simulink library "discretizedSecondOrderIntegrator"  (Simulink 7.6)
settings: Solver=ode45  StartTime=0.0  StopTime=10.0  RelTol=1e-3
undefined symbols (not defined in the file or in its folder): DiscIntNeverNeededParam, LowerLimitX, UpperLimitX
libraries: simulink x28, discretizedSecondOrderIntegrator x12
settings Model: Creator=aselot  LastModifiedBy=aselot

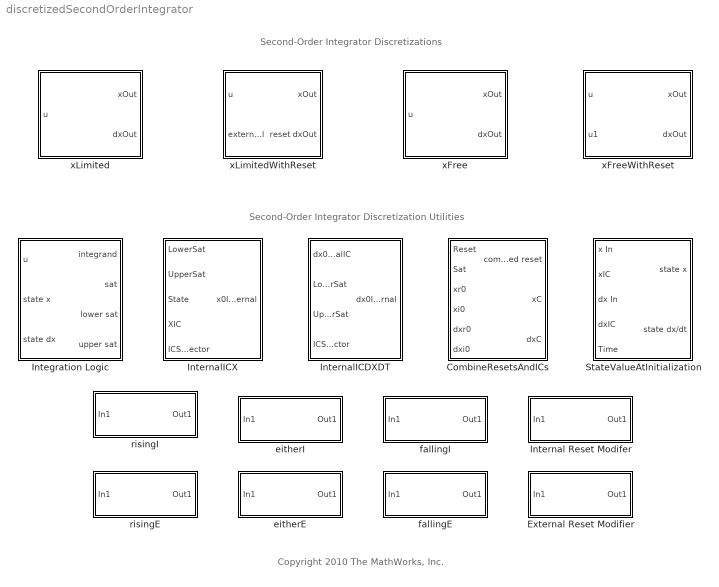
== system discretizedSecondOrderIntegrator ==
  note: Second-Order Integrator Discretizations
  note: Second-Order Integrator Discretization Utilities
  note: Copyright 2010 The MathWorks, Inc.
  CombineResetsAndICs : Subsystem
  External Reset Modifier : Subsystem  BlockChoice=risingE
      settings: TemplateBlock=self  MemberBlocks=eitherE,fallingE,risingE
  Integration Logic : Subsystem
  Internal Reset Modifer : Subsystem  BlockChoice=risingI
      settings: TemplateBlock=self  MemberBlocks=eitherI,fallingI,risingI
  InternalICDXDT : Subsystem  mask{ReinitDXDTwhenXreachesSaturation=off}
      mask prompts: ReinitDXDTwhenXreachesSaturation "Reinitialize dx/dt when x reaches saturation"
      mask init:
      | if strcmp(get_param(gcb, 'ReinitDXDTwhenXreachesSaturation'), 'on')
      |      set_param([gcb '/ReinitializationFlag'], 'Value','1');
      | else
      |     set_param([gcb '/ReinitializationFlag'], 'Value','0');
      | end
  InternalICX : Subsystem
  StateValueAtInitialization : Subsystem
  eitherE : Subsystem
  eitherI : Subsystem
  fallingE : Subsystem
  fallingI : Subsystem
  risingE : Subsystem
  risingI : Subsystem
  xFree : Subsystem  BlockChoice=rising  mask(DiscretizedSecondOrderIntegrator){ICSourceX=internal, ICX=0, LimitX=on, UpperLimitX=1, LowerLimitX=0, ICSourceDXDT=internal, ICDXDT=0, LimitDXDT=off, UpperLimitDXDT=1, LowerLimitDXDT=0, ExternalReset=none, IgnoreStateLimitsAndResetForLinearization=off, ReinitDXDTwhenXreachesSaturation=off, ShowOutput=both, GainValue=1.0, SampleTime=0.1, IntegratorMethod=Integration: Forward Euler}
      mask prompts: ICSourceX "Initial condition source x:"; ICX "Initial condition x:"; LimitX "Limit x"; UpperLimitX "Upper limit x:"; LowerLimitX "Lower limit x:"; ICSourceDXDT "Initial condition source dx/dt:"; ICDXDT "Initial condition dx/dt:"; LimitDXDT "Limit dx/dt"; UpperLimitDXDT "Upper limit dx/dt:"; LowerLimitDXDT "Lower limit dx/dt:"; ExternalReset "External reset"; IgnoreStateLimitsAndResetForLinearization "Ignore state limits and the reset during linearization"; ReinitDXDTwhenXreachesSaturation "Reinitialize dx/dt when x reaches saturation"; ShowOutput "Show output:"; GainValue "Gain value:"; SampleTime "Sample time:"; IntegratorMethod "Integrator method:"
      mask help: A discrete approximation of the continuous Second-Order Integrator block when the states have no limits.
      mask init:
      | configureDiscretizedSecondOrderIntegrator(gcb, 'xFree');
      mask StyleString: popup(internal|external),edit,checkbox,edit,edit,popup(internal|external),edit,checkbox,edit,edit,popup(none),checkbox,checkbox,popup(both|x|dxdt),edit,edit,popup(Integration: Forward Euler|Integration: Backward Euler|Integration: Trapezoidal)
      mask TabNameString: x,x,x,x,x,dx/dt,dx/dt,dx/dt,dx/dt,dx/dt,Attributes,Attributes,Attributes,Attributes,Attributes,Attributes,Attributes
      mask Display:
      | % Draw the icon and label ports for the discretized Second-Order Integrator
      | sIntVariant = 'xFree';
      | 
      | integratorMethod = get_param(gcb, 'IntegratorMethod');
      | 
      | switch(integratorMethod)
      |     case{'Integration: Trapezoidal'}
      |         numerator = 'K^2 Ts^2 (z+1)^2';
      |         text(0.2, 0.6, numerator,'interpreter','tex');
      |         y_line = 0.45;
      |         plot([0.2, 0.8], [y_line,y_line]);
      |         denominator = '4(z-1)^2';
      |         text(0.35, 0.3, denominator,'interpreter','tex');
      |     case{'Integration: Backward Euler'}
      |         numerator = 'K^2 Ts^2 z^2';
      |         text(0.3, 0.63, numerator,'interpreter','tex');
      |         y_line = 0.48;
      |         plot([0.2, 0.8], [y_line,y_line]);
      |         denominator = '(z-1)^2';
      |         text(0.35, 0.33, denominator,'interpreter','tex');
      |     case{'Integration: Forward Euler'}
      |         numerator = 'K^2 Ts^2';
      |         text(0.35, 0.6, numerator,'interpreter','tex');
      |         y_line = 0.45;
      |         plot([0.3, 0.7], [y_line,y_line]);
      |         denominator = '(z-1)^2';
      |         text(0.35, 0.3, denominator,'interpreter','tex');
      | end
      | 
      | portIndex = 1;
      | port_label('input',portIndex,'u');
      | portIndex = portIndex + 1;
      | 
      | if strcmp(sIntVariant, 'xLimitedWithReset') || strcmp(sIntVariant, 'xFreeWithReset')
      |     switch get_param(gcb, 'ExternalReset')
      |         case 'rising'
      |           port_label('input',portIndex,'r');
      |         case 'falling'
      |             port_label('input',portIndex,'f');
      |         case 'either'
      |             port_label('input',portIndex,'e');
      |     end
      |     portIndex = portIndex + 1;
      | end
      | 
      | if strcmp(get_param(gcb,'ICSourceX'),'external')
      |     port_label('input',portIndex,'x_0','texmode','on');
      |     portIndex = portIndex+1;
      | end
      | 
      | if strcmp(get_param(gcb,'ICSourceDXDT'),'external')
      |     port_label('input',portIndex,'dx_0','texmode','on');
      | end
      | 
      | ShowOutput = get_param(gcb,'ShowOutput');
      | 
      | switch ShowOutput
      |     case 'x'
      |         port_label('output',1,'x');
      |     case 'dxdt'
      |         port_label('output',1,'dx');
      |     case 'both'
      |         port_label('output',1,'x');
      |         port_label('output',2,'dx');
      | end
  xFreeWithReset : Subsystem  BlockChoice=rising  mask(DiscretizedSecondOrderIntegrator){ICSourceX=internal, ICX=0, LimitX=on, UpperLimitX=0, LowerLimitX=0, ICSourceDXDT=internal, ICDXDT=0, LimitDXDT=off, UpperLimitDXDT=1, LowerLimitDXDT=0, ExternalReset=rising, IgnoreStateLimitsAndResetForLinearization=off, ReinitDXDTwhenXreachesSaturation=off, ShowOutput=both, GainValue=1.0, SampleTime=0.1, IntegratorMethod=Integration: Forward Euler}
      mask prompts: ICSourceX "Initial condition source x:"; ICX "Initial condition x:"; LimitX "Limit x"; UpperLimitX "Upper limit x:"; LowerLimitX "Lower limit x:"; ICSourceDXDT "Initial condition source dx/dt:"; ICDXDT "Initial condition dx/dt:"; LimitDXDT "Limit dx/dt"; UpperLimitDXDT "Upper limit dx/dt:"; LowerLimitDXDT "Lower limit dx/dt:"; ExternalReset "External reset"; IgnoreStateLimitsAndResetForLinearization "Ignore state limits and the reset during linearization"; ReinitDXDTwhenXreachesSaturation "Reinitialize dx/dt when x reaches saturation"; ShowOutput "Show output:"; GainValue "Gain value:"; SampleTime "Sample time:"; IntegratorMethod "Integrator method:"
      mask help: A discrete approximation of the continuous Second-Order Integrator block when the block has an external reset and the states have no limits.
      mask init:
      | configureDiscretizedSecondOrderIntegrator(gcb, 'xFreeWithReset');
      mask StyleString: popup(internal|external),edit,checkbox,edit,edit,popup(internal|external),edit,checkbox,edit,edit,popup(rising|falling|either),checkbox,checkbox,popup(both|x|dxdt),edit,edit,popup(Integration: Forward Euler|Integration: Backward Euler|Integration: Trapezoidal)
      mask TabNameString: x,x,x,x,x,dx/dt,dx/dt,dx/dt,dx/dt,dx/dt,Attributes,Attributes,Attributes,Attributes,Attributes,Attributes,Attributes
      mask Display:
      | % Draw the icon and label port for the discretized Second-Order Integrator
      | sIntVariant = 'xFreeWithReset';
      | 
      | integratorMethod = get_param(gcb, 'IntegratorMethod');
      | switch(integratorMethod)
      |     case{'Integration: Trapezoidal'}
      |         numerator = 'K^2 Ts^2 (z+1)^2';
      |         text(0.2, 0.6, numerator,'interpreter','tex');
      |         y_line = 0.45;
      |         plot([0.2, 0.8], [y_line,y_line]);
      |         denominator = '4(z-1)^2';
      |         text(0.35, 0.3, denominator,'interpreter','tex');
      |     case{'Integration: Backward Euler'}
      |         numerator = 'K^2 Ts^2 z^2';
      |         text(0.3, 0.63, numerator,'interpreter','tex');
      |         y_line = 0.48;
      |         plot([0.2, 0.8], [y_line,y_line]);
      |         denominator = '(z-1)^2';
      |         text(0.35, 0.33, denominator,'interpreter','tex');
      |     case{'Integration: Forward Euler'}
      |         numerator = 'K^2 Ts^2';
      |         text(0.35, 0.6, numerator,'interpreter','tex');
      |         y_line = 0.45;
      |         plot([0.3, 0.7], [y_line,y_line]);
      |         denominator = '(z-1)^2';
      |         text(0.35, 0.3, denominator,'interpreter','tex');
      | end
      | 
      | portIndex = 1;
      | port_label('input',portIndex,'u');
      | portIndex = portIndex + 1;
      | 
      | if strcmp(sIntVariant, 'xLimitedWithReset') || strcmp(sIntVariant, 'xFreeWithReset')
      |     switch get_param(gcb, 'ExternalReset')
      |         case 'rising'
      |           port_label('input',portIndex,'r');
      |         case 'falling'
      |             port_label('input',portIndex,'f');
      |         case 'either'
      |             port_label('input',portIndex,'e');
      |     end
      |     portIndex = portIndex + 1;
      | end
      | 
      | if strcmp(get_param(gcb,'ICSourceX'),'external')
      |     port_label('input',portIndex,'x_0','texmode','on');
      |     portIndex = portIndex+1;
      | end
      | 
      | if strcmp(get_param(gcb,'ICSourceDXDT'),'external')
      |     port_label('input',portIndex,'dx_0','texmode','on');
      | end
      | 
      | ShowOutput = get_param(gcb,'ShowOutput');
      | 
      | switch ShowOutput
      |     case 'x'
      |         port_label('output',1,'x');
      |     case 'dxdt'
      |         port_label('output',1,'dx');
      |     case 'both'
      |         port_label('output',1,'x');
      |         port_label('output',2,'dx');
      | end
  xLimited : Subsystem  BlockChoice=rising  mask(DiscretizedSecondOrderIntegrator){ICSourceX=internal, ICX=0, LimitX=on, UpperLimitX=1, LowerLimitX=0, ICSourceDXDT=internal, ICDXDT=0, LimitDXDT=off, UpperLimitDXDT=1, LowerLimitDXDT=0, ExternalReset=none, IgnoreStateLimitsAndResetForLinearization=off, ReinitDXDTwhenXreachesSaturation=off, ShowOutput=both, GainValue=1.0, SampleTime=0.1, IntegratorMethod=Integration: Forward Euler}
      mask prompts: ICSourceX "Initial condition source x:"; ICX "Initial condition x:"; LimitX "Limit x"; UpperLimitX "Upper limit x:"; LowerLimitX "Lower limit x:"; ICSourceDXDT "Initial condition source dx/dt:"; ICDXDT "Initial condition dx/dt:"; LimitDXDT "Limit dx/dt"; UpperLimitDXDT "Upper limit dx/dt:"; LowerLimitDXDT "Lower limit dx/dt:"; ExternalReset "External reset"; IgnoreStateLimitsAndResetForLinearization "Ignore state limits and the reset during linearization"; ReinitDXDTwhenXreachesSaturation "Reinitialize dx/dt when x reaches saturation"; ShowOutput "Show output:"; GainValue "Gain value:"; SampleTime "Sample time:"; IntegratorMethod "Integrator method:"
      mask help: A discrete approximation of the continuous Second-Order Integrator block when the state x has limits.
      mask init:
      | configureDiscretizedSecondOrderIntegrator(gcb, 'xLimited');
      mask StyleString: popup(internal|external),edit,checkbox,edit,edit,popup(internal|external),edit,checkbox,edit,edit,popup(none),checkbox,checkbox,popup(both|x|dxdt),edit,edit,popup(Integration: Forward Euler|Integration: Backward Euler|Integration: Trapezoidal)
      mask TabNameString: x,x,x,x,x,dx/dt,dx/dt,dx/dt,dx/dt,dx/dt,Attributes,Attributes,Attributes,Attributes,Attributes,Attributes,Attributes
      mask Display:
      | % Draw the icon and label ports for the discretized Second-Order Integrator
      | sIntVariant = 'xLimited';
      | numerator = 'K^2 Ts^2';
      | text(0.35, 0.6, numerator,'interpreter','tex');
      | y_line = 0.45;
      | plot([0.3, 0.7], [y_line,y_line]);
      | denominator = '(z-1)^2';
      | text(0.35, 0.3, denominator,'interpreter','tex');
      | 
      | 
      | portIndex = 1;
      | port_label('input',portIndex,'u');
      | portIndex = portIndex + 1;
      | 
      | if strcmp(sIntVariant, 'xLimitedWithReset') || strcmp(sIntVariant, 'xFreeWithReset')
      |     switch get_param(gcb, 'ExternalReset')
      |         case 'rising'
      |           port_label('input',portIndex,'r');
      |         case 'falling'
      |             port_label('input',portIndex,'f');
      |         case 'either'
      |             port_label('input',portIndex,'e');
      |     end
      |     portIndex = portIndex + 1;
      | end
      | 
      | if strcmp(get_param(gcb,'ICSourceX'),'external')
      |     port_label('input',portIndex,'x_0','texmode','on');
      |     portIndex = portIndex+1;
      | end
      | 
      | if strcmp(get_param(gcb,'ICSourceDXDT'),'external')
      |     port_label('input',portIndex,'dx_0','texmode','on');
      | end
      | 
      | ShowOutput = get_param(gcb,'ShowOutput');
      | 
      | switch ShowOutput
      |     case 'x'
      |         port_label('output',1,'x');
      |     case 'dxdt'
      |         port_label('output',1,'dx');
      |     case 'both'
      |         port_label('output',1,'x');
      |         port_label('output',2,'dx');
      | end
  xLimitedWithReset : Subsystem  BlockChoice=rising  mask(DiscretizedSecondOrderIntegrator){ICSourceX=internal, ICX=0, LimitX=on, UpperLimitX=1, LowerLimitX=0, ICSourceDXDT=internal, ICDXDT=0, LimitDXDT=off, UpperLimitDXDT=1, LowerLimitDXDT=0, ExternalReset=rising, IgnoreStateLimitsAndResetForLinearization=off, ReinitDXDTwhenXreachesSaturation=off, ShowOutput=both, GainValue=1.0, SampleTime=0.1, IntegratorMethod=Integration: Forward Euler}
      mask prompts: ICSourceX "Initial condition source x:"; ICX "Initial condition x:"; LimitX "Limit x"; UpperLimitX "Upper limit x:"; LowerLimitX "Lower limit x:"; ICSourceDXDT "Initial condition source dx/dt"; ICDXDT "Initial condition dx/dt:"; LimitDXDT "Limit dx/dt"; UpperLimitDXDT "Upper limit dx/dt:"; LowerLimitDXDT "Lower limit dx/dt:"; ExternalReset "External reset"; IgnoreStateLimitsAndResetForLinearization "Ignore state limits and the reset during linearization"; ReinitDXDTwhenXreachesSaturation "Reinitialize dx/dt when x reaches saturation"; ShowOutput "Show output:"; GainValue "Gain value:"; SampleTime "Sample time:"; IntegratorMethod "Integrator method:"
      mask help: A discrete approximation of the continuous Second-Order Integrator block when the block has an external reset and the state x has limits.
      mask init:
      | configureDiscretizedSecondOrderIntegrator(gcb, 'xLimitedWithReset');
      mask StyleString: popup(internal|external),edit,checkbox,edit,edit,popup(internal|external),edit,checkbox,edit,edit,popup(rising|falling|either),checkbox,checkbox,popup(both|x|dxdt),edit,edit,popup(Integration: Forward Euler|Integration: Backward Euler|Integration: Trapezoidal)
      mask TabNameString: x,x,x,x,x,dx/dt,dx/dt,dx/dt,dx/dt,dx/dt,Attributes,Attributes,Attributes,Attributes,Attributes,Attributes,Attributes
      mask Display:
      | % Draw the icon and label ports for the discretized Second-Order Integrator
      | sIntVariant = 'xLimitedWithReset';
      | 
      | numerator = 'K^2 Ts^2';
      | text(0.35, 0.6, numerator,'interpreter','tex');
      | y_line = 0.45;
      | plot([0.3, 0.7], [y_line,y_line]);
      | denominator = '(z-1)^2';
      | text(0.35, 0.3, denominator,'interpreter','tex');
      | 
      | 
      | portIndex = 1;
      | port_label('input',portIndex,'u');
      | portIndex = portIndex + 1;
      | 
      | if strcmp(sIntVariant, 'xLimitedWithReset') || strcmp(sIntVariant, 'xFreeWithReset')
      |     switch get_param(gcb, 'ExternalReset')
      |         case 'rising'
      |             port_label('input',portIndex,'r');
      |         case 'falling'
      |             port_label('input',portIndex,'f');
      |         case 'either'
      |             port_label('input',portIndex,'e');
      |     end
      |     portIndex = portIndex + 1;
      | end
      | 
      | if strcmp(get_param(gcb,'ICSourceX'),'external')
      |     port_label('input',portIndex,'x_0','texmode','on');
      |     portIndex = portIndex+1;
      | end
      | 
      | if strcmp(get_param(gcb,'ICSourceDXDT'),'external')
      |     port_label('input',portIndex,'dx_0','texmode','on');
      | end
      | 
      | ShowOutput = get_param(gcb,'ShowOutput');
      | 
      | switch ShowOutput
      |     case 'x'
      |         port_label('output',1,'x');
      |     case 'dxdt'
      |         port_label('output',1,'dx');
      |     case 'both'
      |         port_label('output',1,'x');
      |         port_label('output',2,'dx');
      | end

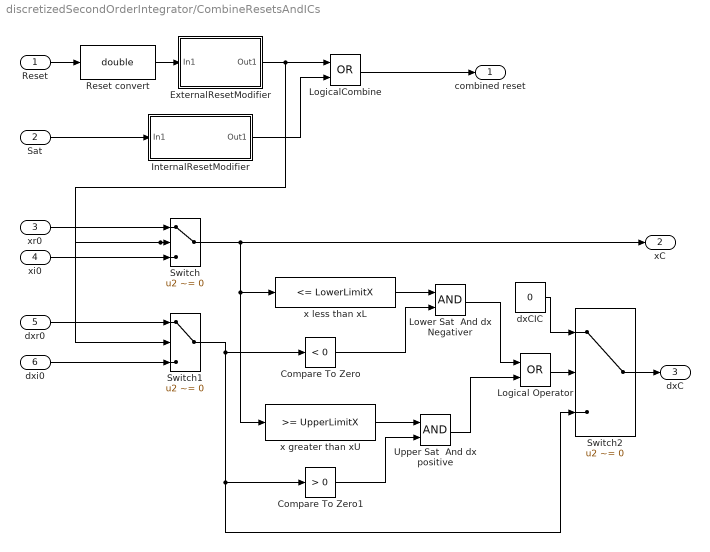
== system discretizedSecondOrderIntegrator/CombineResetsAndICs ==
  "Reset " : Inport  OutDataType=fixdt(1, 16)  OutScaling=2^0
  Sat : Inport  Port=2  OutDataType=fixdt(1, 16)  OutScaling=2^0
  xr0 : Inport  Port=3  OutDataType=fixdt(1, 16)  OutScaling=2^0
  xi0 : Inport  Port=4  OutDataType=fixdt(1, 16)  OutScaling=2^0
  dxr0 : Inport  Port=5  OutDataType=fixdt(1, 16)  OutScaling=2^0
  dxi0 : Inport  Port=6  OutDataType=fixdt(1, 16)  OutScaling=2^0
  Compare To Zero : simulink/Logic and Bit Operations/Compare To Zero  SystemSampleTime=-1  relop=<  LogicOutDataTypeMode=boolean
  Compare To Zero1 : simulink/Logic and Bit Operations/Compare To Zero  SystemSampleTime=-1  relop=>  LogicOutDataTypeMode=boolean
  ExternalResetModifier : Subsystem  BlockChoice=risingE
      settings: AttributesFormatString=%<BlockChoice>  TemplateBlock=discretizedSecondOrderIntegrator/External Reset Modifier  MemberBlocks=eitherE,fallingE,risingE
  InternalResetModifier : Subsystem  BlockChoice=risingI
      settings: AttributesFormatString=%<BlockChoice>  TemplateBlock=discretizedSecondOrderIntegrator/Internal Reset Modifer  MemberBlocks=eitherI,fallingI,risingI
  Logical Operator : Logic  Operator=OR  AllPortsSameDT=off  OutDataTypeMode=boolean  LogicDataType=fixdt(0, 8)  OutDataTypeStr=boolean
  LogicalCombine : Logic  Operator=OR  AllPortsSameDT=off  OutDataTypeMode=boolean  LogicDataType=fixdt(0, 8)  OutDataTypeStr=boolean
  Lower Sat  And dx Negativer : Logic  AllPortsSameDT=off  OutDataTypeMode=boolean  LogicDataType=fixdt(0, 8)  OutDataTypeStr=boolean
  Reset convert : DataTypeConversion  OutDataTypeMode=double  OutDataType=fixdt(1, 16)  OutScaling=2^0  OutDataTypeStr=double
  Switch : Switch  Criteria=u2 ~= 0  OutDataType=fixdt(1, 16)  OutScaling=2^0
  Switch1 : Switch  Criteria=u2 ~= 0  OutDataType=fixdt(1, 16)  OutScaling=2^0
  Switch2 : Switch  Criteria=u2 ~= 0  OutDataType=fixdt(1, 16)  OutScaling=2^0
  Upper Sat  And dx positive : Logic  AllPortsSameDT=off  OutDataTypeMode=boolean  LogicDataType=fixdt(0, 8)  OutDataTypeStr=boolean
  dxCIC : Constant  Value=0  OutDataType=fixdt(1, 16)  OutScaling=2^0
  x greater than xU : simulink/Logic and Bit Operations/Compare To Constant  SystemSampleTime=-1  relop=>=  const=UpperLimitX  LogicOutDataTypeMode=boolean
  x less than xL : simulink/Logic and Bit Operations/Compare To Constant  SystemSampleTime=-1  relop=<=  const=LowerLimitX  LogicOutDataTypeMode=boolean
  combined reset : Outport  OutDataType=fixdt(1, 16)  OutScaling=2^0
  xC : Outport  Port=2  OutDataType=fixdt(1, 16)  OutScaling=2^0
  dxC : Outport  Port=3  OutDataType=fixdt(1, 16)  OutScaling=2^0
  wires:
  Sat/1 -> InternalResetModifier/1(In1)
  dxi0/1 -> Switch1/3
  dxr0/1 -> Switch1/1
  LogicalCombine/1 -> combined reset/1
  "Reset "/1 -> Reset convert/1
  ExternalResetModifier/1(Out1) -> Switch1/2, Switch/2, LogicalCombine/1
  Reset convert/1 -> ExternalResetModifier/1(In1)
  xr0/1 -> Switch/1
  xi0/1 -> Switch/3
  Logical Operator/1 -> Switch2/2
  Switch2/1 -> dxC/1
  Switch1/1 -> Switch2/3, Compare To Zero1/1, Compare To Zero/1
  Switch/1 -> xC/1, x less than xL/1, x greater than xU/1
  dxCIC/1 -> Switch2/1
  Lower Sat  And dx Negativer/1 -> Logical Operator/1
  Upper Sat  And dx positive/1 -> Logical Operator/2
  x less than xL/1 -> Lower Sat  And dx Negativer/1
  x greater than xU/1 -> Upper Sat  And dx positive/1
  Compare To Zero1/1 -> Upper Sat  And dx positive/2
  Compare To Zero/1 -> Lower Sat  And dx Negativer/2
  InternalResetModifier/1(Out1) -> LogicalCombine/2

== system discretizedSecondOrderIntegrator/External Reset Modifier ==
  In1 : Inport
  risingE : discretizedSecondOrderIntegrator/risingE  SystemSampleTime=-1
  Out1 : Outport
  wires:
  In1/1 -> risingE/1
  risingE/1 -> Out1/1

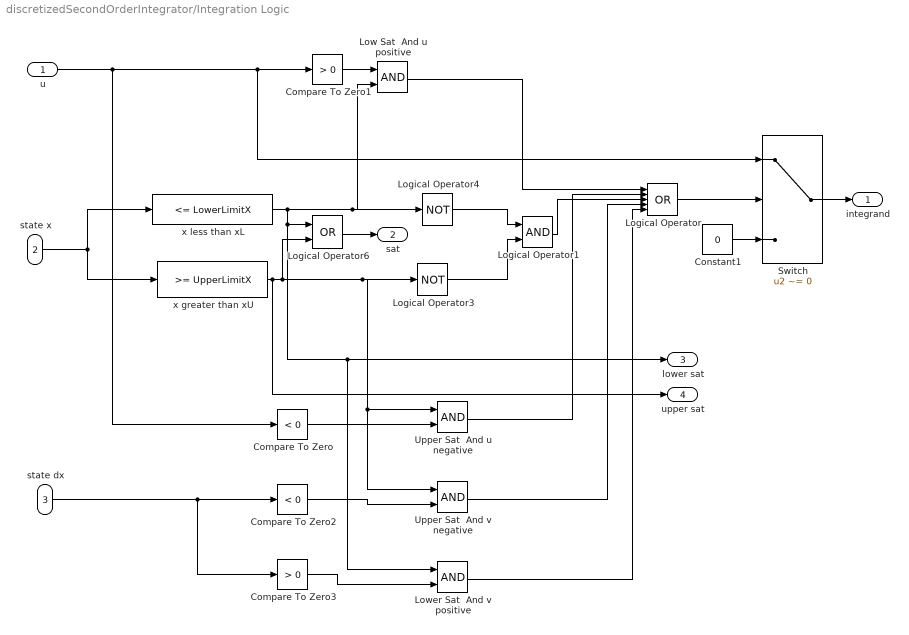
== system discretizedSecondOrderIntegrator/Integration Logic ==
  u : Inport
  state x : Inport  Port=2
  state dx : Inport  Port=3
  Compare To Zero : simulink/Logic and Bit Operations/Compare To Zero  SystemSampleTime=-1  relop=<  LogicOutDataTypeMode=boolean
  Compare To Zero1 : simulink/Logic and Bit Operations/Compare To Zero  SystemSampleTime=-1  relop=>  LogicOutDataTypeMode=boolean
  Compare To Zero2 : simulink/Logic and Bit Operations/Compare To Zero  SystemSampleTime=-1  relop=<  LogicOutDataTypeMode=boolean
  Compare To Zero3 : simulink/Logic and Bit Operations/Compare To Zero  SystemSampleTime=-1  relop=>  LogicOutDataTypeMode=boolean
  Constant1 : Constant  Value=0  OutDataType=fixdt(1, 16)  OutScaling=2^0
  Logical Operator : Logic  Operator=OR  Inputs=5  AllPortsSameDT=off  OutDataTypeMode=boolean  LogicDataType=fixdt(0, 8)  OutDataTypeStr=boolean
  Logical Operator1 : Logic  AllPortsSameDT=off  OutDataTypeMode=boolean  LogicDataType=fixdt(0, 8)  OutDataTypeStr=boolean
  Logical Operator3 : Logic  Operator=NOT  AllPortsSameDT=off  OutDataTypeMode=boolean  LogicDataType=fixdt(0, 8)  OutDataTypeStr=boolean
  Logical Operator4 : Logic  Operator=NOT  AllPortsSameDT=off  OutDataTypeMode=boolean  LogicDataType=fixdt(0, 8)  OutDataTypeStr=boolean
  Logical Operator6 : Logic  Operator=OR  AllPortsSameDT=off  OutDataTypeMode=boolean  LogicDataType=fixdt(0, 8)  OutDataTypeStr=boolean
  Low Sat  And u positive : Logic  AllPortsSameDT=off  OutDataTypeMode=boolean  LogicDataType=fixdt(0, 8)  OutDataTypeStr=boolean
  Lower Sat  And v positive : Logic  AllPortsSameDT=off  OutDataTypeMode=boolean  LogicDataType=fixdt(0, 8)  OutDataTypeStr=boolean
  Switch : Switch  Criteria=u2 ~= 0  OutDataType=fixdt(1, 16)  OutScaling=2^0
  Upper Sat  And u negative : Logic  AllPortsSameDT=off  OutDataTypeMode=boolean  LogicDataType=fixdt(0, 8)  OutDataTypeStr=boolean
  Upper Sat  And v negative : Logic  AllPortsSameDT=off  OutDataTypeMode=boolean  LogicDataType=fixdt(0, 8)  OutDataTypeStr=boolean
  x greater than xU : simulink/Logic and Bit Operations/Compare To Constant  SystemSampleTime=-1  relop=>=  const=UpperLimitX  LogicOutDataTypeMode=boolean
  x less than xL : simulink/Logic and Bit Operations/Compare To Constant  SystemSampleTime=-1  relop=<=  const=LowerLimitX  LogicOutDataTypeMode=boolean
  integrand : Outport
  sat : Outport  Port=2
  lower sat : Outport  Port=3
  upper sat : Outport  Port=4
  wires:
  Logical Operator6/1 -> sat/1
  state x/1 -> x less than xL/1, x greater than xU/1
  u/1 -> Compare To Zero/1, Compare To Zero1/1, Switch/1
  Switch/1 -> integrand/1
  Logical Operator/1 -> Switch/2
  Constant1/1 -> Switch/3
  Logical Operator4/1 -> Logical Operator1/1
  Logical Operator3/1 -> Logical Operator1/2
  Compare To Zero1/1 -> Low Sat  And u positive/1
  x less than xL/1 -> Low Sat  And u positive/2, Logical Operator4/1, Logical Operator6/1, lower sat/1, Lower Sat  And v positive/1
  Low Sat  And u positive/1 -> Logical Operator/1
  x greater than xU/1 -> Logical Operator6/2, Logical Operator3/1, Upper Sat  And u negative/1, Upper Sat  And v negative/1, upper sat/1
  Compare To Zero/1 -> Upper Sat  And u negative/2
  Upper Sat  And u negative/1 -> Logical Operator/2
  Logical Operator1/1 -> Logical Operator/3
  state dx/1 -> Compare To Zero2/1, Compare To Zero3/1
  Compare To Zero2/1 -> Upper Sat  And v negative/2
  Compare To Zero3/1 -> Lower Sat  And v positive/2
  Upper Sat  And v negative/1 -> Logical Operator/4
  Lower Sat  And v positive/1 -> Logical Operator/5

== system discretizedSecondOrderIntegrator/Internal Reset Modifer ==
  In1 : Inport
  risingI : discretizedSecondOrderIntegrator/risingI  SystemSampleTime=-1
  Out1 : Outport
  wires:
  In1/1 -> risingI/1
  risingI/1 -> Out1/1

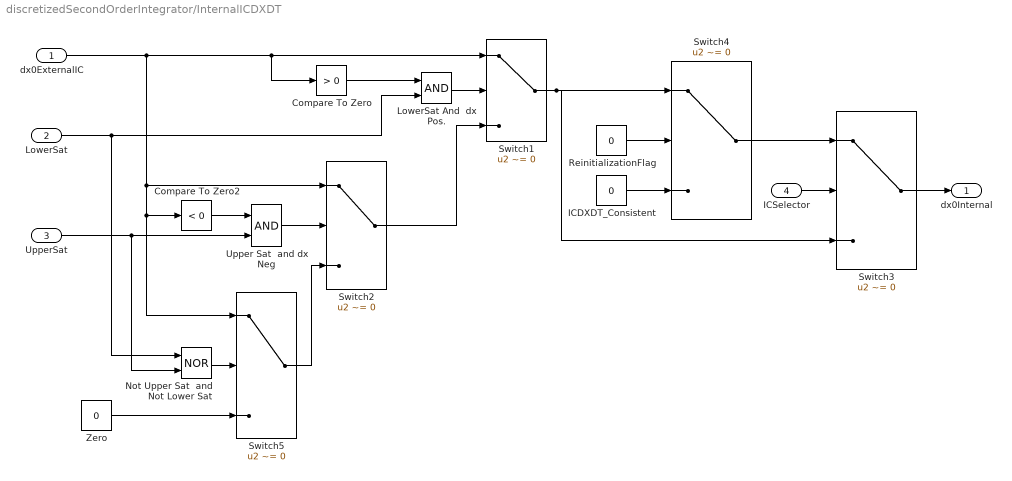
== system discretizedSecondOrderIntegrator/InternalICDXDT ==
  dx0ExternalIC : Inport
  LowerSat : Inport  Port=2
  UpperSat : Inport  Port=3
  ICSelector : Inport  Port=4
  Compare To Zero : simulink/Logic and Bit Operations/Compare To Zero  SystemSampleTime=-1  relop=>  LogicOutDataTypeMode=boolean
  Compare To Zero2 : simulink/Logic and Bit Operations/Compare To Zero  SystemSampleTime=-1  relop=<  LogicOutDataTypeMode=boolean
  ICDXDT_Consistent : Constant  Value=0  OutDataType=fixdt(1, 16)  OutScaling=2^0
  LowerSat And  dx Pos. : Logic  AllPortsSameDT=off  OutDataTypeMode=boolean  LogicDataType=fixdt(0, 8)  OutDataTypeStr=boolean
  Not Upper Sat  and Not Lower Sat : Logic  Operator=NOR  AllPortsSameDT=off  OutDataTypeMode=boolean  LogicDataType=fixdt(0, 8)  OutDataTypeStr=boolean
  ReinitializationFlag : Constant  Value=0  OutDataType=fixdt(1, 16)  OutScaling=2^0
  Switch{1..5} (5 alike) : Switch  Criteria=u2 ~= 0  OutDataType=fixdt(1, 16)  OutScaling=2^0
  Upper Sat  and dx Neg : Logic  AllPortsSameDT=off  OutDataTypeMode=boolean  LogicDataType=fixdt(0, 8)  OutDataTypeStr=boolean
  Zero : Constant  Value=0  OutDataType=fixdt(1, 16)  OutScaling=2^0
  dx0Internal : Outport
  wires:
  ICSelector/1 -> Switch3/2
  Upper Sat  and dx Neg/1 -> Switch2/2
  LowerSat And  dx Pos./1 -> Switch1/2
  Compare To Zero/1 -> LowerSat And  dx Pos./1
  LowerSat/1 -> LowerSat And  dx Pos./2, Not Upper Sat  and Not Lower Sat/1
  Switch2/1 -> Switch1/3
  UpperSat/1 -> Upper Sat  and dx Neg/2, Not Upper Sat  and Not Lower Sat/2
  Compare To Zero2/1 -> Upper Sat  and dx Neg/1
  Switch1/1 -> Switch4/1, Switch3/3
  Switch3/1 -> dx0Internal/1
  ReinitializationFlag/1 -> Switch4/2
  ICDXDT_Consistent/1 -> Switch4/3
  dx0ExternalIC/1 -> Switch2/1, Switch5/1, Compare To Zero2/1, Compare To Zero/1, Switch1/1
  Switch4/1 -> Switch3/1
  Zero/1 -> Switch5/3
  Switch5/1 -> Switch2/3
  Not Upper Sat  and Not Lower Sat/1 -> Switch5/2

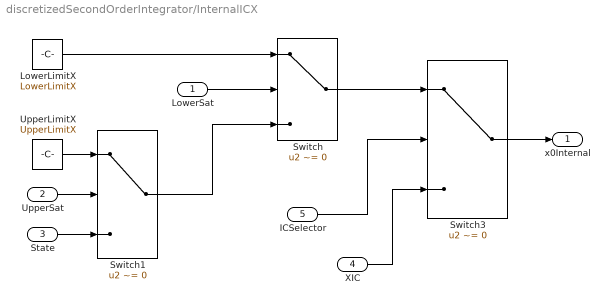
== system discretizedSecondOrderIntegrator/InternalICX ==
  LowerSat : Inport
  UpperSat : Inport  Port=2
  State : Inport  Port=3
  XIC : Inport  Port=4
  ICSelector : Inport  Port=5
  LowerLimitX : Constant  Value=LowerLimitX  OutDataType=fixdt(1, 16)  OutScaling=2^0
  Switch : Switch  Criteria=u2 ~= 0  OutDataType=fixdt(1, 16)  OutScaling=2^0
  Switch1 : Switch  Criteria=u2 ~= 0  OutDataType=fixdt(1, 16)  OutScaling=2^0
  Switch3 : Switch  Criteria=u2 ~= 0  OutDataType=fixdt(1, 16)  OutScaling=2^0
  UpperLimitX : Constant  Value=UpperLimitX  OutDataType=fixdt(1, 16)  OutScaling=2^0
  x0Internal : Outport
  wires:
  ICSelector/1 -> Switch3/2
  XIC/1 -> Switch3/3
  Switch3/1 -> x0Internal/1
  UpperLimitX/1 -> Switch1/1
  Switch/1 -> Switch3/1
  LowerLimitX/1 -> Switch/1
  LowerSat/1 -> Switch/2
  UpperSat/1 -> Switch1/2
  Switch1/1 -> Switch/3
  State/1 -> Switch1/3

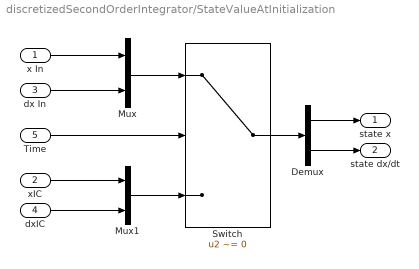
== system discretizedSecondOrderIntegrator/StateValueAtInitialization ==
  x In : Inport
  xIC : Inport  Port=2
  dx In : Inport  Port=3
  dxIC : Inport  Port=4
  Time : Inport  Port=5
  Demux : Demux  Outputs=2
  Mux : Mux  Inputs=2
  Mux1 : Mux  Inputs=2
  Switch : Switch  Criteria=u2 ~= 0  OutDataType=fixdt(1, 16)  OutScaling=2^0
  state x : Outport
  state dx/dt : Outport  Port=2
  wires:
  Time/1 -> Switch/2
  x In/1 -> Mux/1
  dx In/1 -> Mux/2
  Mux/1 -> Switch/1
  xIC/1 -> Mux1/1
  dxIC/1 -> Mux1/2
  Mux1/1 -> Switch/3
  Switch/1 -> Demux/1
  Demux/1 -> state x/1
  Demux/2 -> state dx/dt/1

== system discretizedSecondOrderIntegrator/eitherE ==
  In1 : Inport  OutDataType=fixdt(1, 16)  OutScaling=2^0
  Detect Change : simulink/Logic and Bit Operations/Detect Change  SystemSampleTime=-1  vinit=0
  Hit  Crossing : HitCross
  Out1 : Outport  OutDataType=fixdt(1, 16)  OutScaling=2^0
  wires:
  Hit  Crossing/1 -> Detect Change/1
  In1/1 -> Hit  Crossing/1
  Detect Change/1 -> Out1/1

== system discretizedSecondOrderIntegrator/eitherI ==
  In1 : Inport  OutDataType=fixdt(1, 16)  OutScaling=2^0
  either : simulink/Logic and Bit Operations/Detect Rise Positive  SystemSampleTime=-1  vinit=0
  Out1 : Outport  OutDataType=fixdt(1, 16)  OutScaling=2^0
  wires:
  either/1 -> Out1/1
  In1/1 -> either/1

== system discretizedSecondOrderIntegrator/fallingE ==
  In1 : Inport  OutDataType=fixdt(1, 16)  OutScaling=2^0
  Compare To Zero : simulink/Logic and Bit Operations/Compare To Zero  SystemSampleTime=-1  relop=>=  LogicOutDataTypeMode=uint8
  Detect Decrease : simulink/Logic and Bit Operations/Detect Decrease  SystemSampleTime=-1  vinit=0.0
  Out1 : Outport  OutDataType=fixdt(1, 16)  OutScaling=2^0
  wires:
  In1/1 -> Compare To Zero/1
  Detect Decrease/1 -> Out1/1
  Compare To Zero/1 -> Detect Decrease/1

== system discretizedSecondOrderIntegrator/fallingI ==
  In1 : Inport  OutDataType=fixdt(1, 16)  OutScaling=2^0
  Detect Decrease : simulink/Logic and Bit Operations/Detect Decrease  SystemSampleTime=-1  vinit=0.0
  falling : Logic  Operator=NOT  AllPortsSameDT=off  OutDataTypeMode=boolean  LogicDataType=fixdt(0, 8)  OutDataTypeStr=boolean
  Out1 : Outport  OutDataType=fixdt(1, 16)  OutScaling=2^0
  wires:
  falling/1 -> Detect Decrease/1
  In1/1 -> falling/1
  Detect Decrease/1 -> Out1/1

== system discretizedSecondOrderIntegrator/risingE ==
  In1 : Inport  OutDataType=fixdt(1, 16)  OutScaling=2^0
  Compare To Zero : simulink/Logic and Bit Operations/Compare To Zero  SystemSampleTime=-1  relop=>=  LogicOutDataTypeMode=uint8
  Detect Increase : simulink/Logic and Bit Operations/Detect Increase  SystemSampleTime=-1  vinit=0.0
  Out1 : Outport  OutDataType=fixdt(1, 16)  OutScaling=2^0
  wires:
  In1/1 -> Compare To Zero/1
  Detect Increase/1 -> Out1/1
  Compare To Zero/1 -> Detect Increase/1

== system discretizedSecondOrderIntegrator/risingI ==
  In1 : Inport  OutDataType=fixdt(1, 16)  OutScaling=2^0
  Detect Increase : simulink/Logic and Bit Operations/Detect Increase  SystemSampleTime=-1  vinit=0.0
  Out1 : Outport  OutDataType=fixdt(1, 16)  OutScaling=2^0
  wires:
  In1/1 -> Detect Increase/1
  Detect Increase/1 -> Out1/1

== system discretizedSecondOrderIntegrator/xFree ==
  u : Inport
  dx0 : Constant  Value=ICDXDT
  dxdt : DiscreteIntegrator  gainval=GainValue  InitialConditionSource=external  InitialCondition=ICDXDT  SampleTime=SampleTime  OutDataType=fixdt(1, 16)  OutScaling=2^0  UpperSaturationLimit=UpperLimitDXDT  LowerSaturationLimit=LowerLimitDXDT  ICPrevOutput=DiscIntNeverNeededParam  ICPrevScaledInput=DiscIntNeverNeededParam
  x : DiscreteIntegrator  gainval=GainValue  InitialConditionSource=external  InitialCondition=ICX  SampleTime=SampleTime  OutDataType=fixdt(1, 16)  OutScaling=2^0  UpperSaturationLimit=UpperLimitX  LowerSaturationLimit=LowerLimitX  ICPrevOutput=DiscIntNeverNeededParam  ICPrevScaledInput=DiscIntNeverNeededParam
  x0 : Constant  Value=ICX
  xOut : Outport
  dxOut : Outport  Port=2
  wires:
  u/1 -> dxdt/1
  x/1 -> xOut/1
  x0/1 -> x/2
  dx0/1 -> dxdt/2
  dxdt/1 -> x/1, dxOut/1

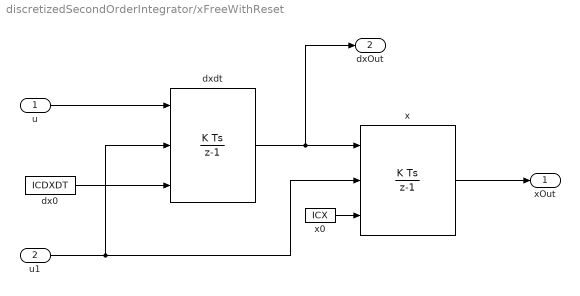
== system discretizedSecondOrderIntegrator/xFreeWithReset ==
  u : Inport
  u1 : Inport  Port=2
  dx0 : Constant  Value=ICDXDT
  dxdt : DiscreteIntegrator  gainval=GainValue  ExternalReset=rising  InitialConditionSource=external  InitialCondition=ICDXDT  SampleTime=SampleTime  OutDataType=fixdt(1, 16)  OutScaling=2^0  UpperSaturationLimit=UpperLimitDXDT  LowerSaturationLimit=LowerLimitDXDT  ICPrevOutput=DiscIntNeverNeededParam  ICPrevScaledInput=DiscIntNeverNeededParam
  x : DiscreteIntegrator  gainval=GainValue  ExternalReset=rising  InitialConditionSource=external  InitialCondition=ICX  SampleTime=SampleTime  OutDataType=fixdt(1, 16)  OutScaling=2^0  UpperSaturationLimit=UpperLimitX  LowerSaturationLimit=LowerLimitX  ICPrevOutput=DiscIntNeverNeededParam  ICPrevScaledInput=DiscIntNeverNeededParam
  x0 : Constant  Value=ICX
  xOut : Outport
  dxOut : Outport  Port=2
  wires:
  dxdt/1 -> dxOut/1, x/1
  dx0/1 -> dxdt/3
  x0/1 -> x/3
  x/1 -> xOut/1
  u/1 -> dxdt/1
  u1/1 -> dxdt/2, x/2

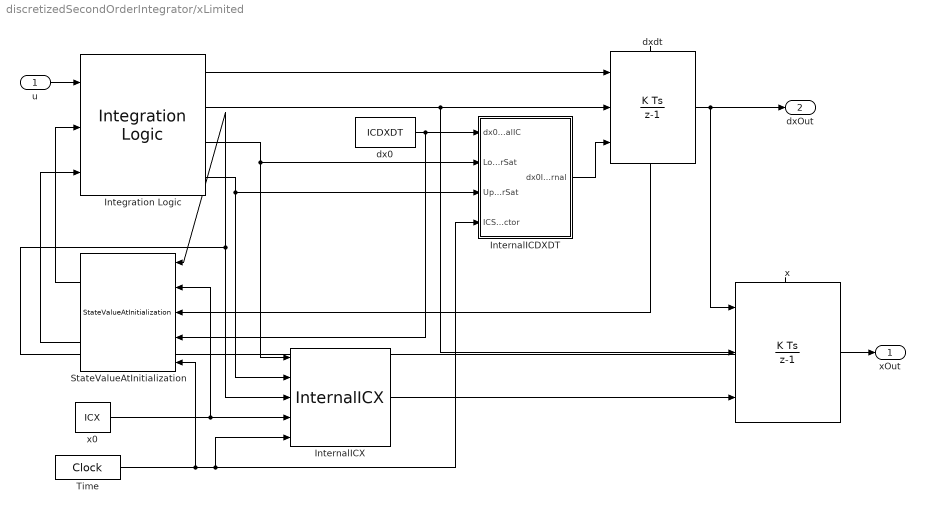
== system discretizedSecondOrderIntegrator/xLimited ==
  u : Inport
  Integration Logic : discretizedSecondOrderIntegrator/Integration Logic  SystemSampleTime=-1
  InternalICDXDT : Subsystem  mask{ReinitDXDTwhenXreachesSaturation=off}
      mask prompts: ReinitDXDTwhenXreachesSaturation "Reinitialize dx/dt when x reaches saturation"
      mask init:
      | if strcmp(get_param(gcb, 'ReinitDXDTwhenXreachesSaturation'), 'on')
      |      set_param([gcb '/ReinitializationFlag'], 'Value','1');
      | else
      |     set_param([gcb '/ReinitializationFlag'], 'Value','0');
      | end
  InternalICX : discretizedSecondOrderIntegrator/InternalICX  SystemSampleTime=-1
  StateValueAtInitialization : discretizedSecondOrderIntegrator/StateValueAtInitialization  SystemSampleTime=-1
  Time : DigitalClock  SampleTime=SampleTime
  dx0 : Constant  Value=ICDXDT
  dxdt : DiscreteIntegrator  gainval=GainValue  ExternalReset=rising  InitialConditionSource=external  InitialCondition=ICDXDT  SampleTime=SampleTime  OutDataType=fixdt(1, 16)  OutScaling=2^0  UpperSaturationLimit=UpperLimitDXDT  LowerSaturationLimit=LowerLimitDXDT  ShowStatePort=on  ICPrevOutput=DiscIntNeverNeededParam  ICPrevScaledInput=DiscIntNeverNeededParam
  x : DiscreteIntegrator  gainval=GainValue  ExternalReset=rising  InitialConditionSource=external  InitialCondition=ICX  SampleTime=SampleTime  OutDataType=fixdt(1, 16)  OutScaling=2^0  LimitOutput=on  UpperSaturationLimit=UpperLimitX  LowerSaturationLimit=LowerLimitX  ShowStatePort=on  StateIdentifier=StateNameX  ICPrevOutput=DiscIntNeverNeededParam  ICPrevScaledInput=DiscIntNeverNeededParam
  x0 : Constant  Value=ICX
  xOut : Outport
  dxOut : Outport  Port=2
  wires:
  Integration Logic/1 -> dxdt/1
  u/1 -> Integration Logic/1
  Time/1 -> InternalICX/5, InternalICDXDT/4(ICSelector), StateValueAtInitialization/5
  InternalICX/1 -> x/3
  Integration Logic/2 -> x/2, dxdt/2
  Integration Logic/4 -> InternalICX/2, InternalICDXDT/3(UpperSat)
  Integration Logic/3 -> InternalICX/1, InternalICDXDT/2(LowerSat)
  x/State -> InternalICX/3, StateValueAtInitialization/1
  x0/1 -> InternalICX/4, StateValueAtInitialization/2
  dxdt/1 -> dxOut/1, x/1
  x/1 -> xOut/1
  dx0/1 -> StateValueAtInitialization/4, InternalICDXDT/1(dx0ExternalIC)
  StateValueAtInitialization/1 -> Integration Logic/2
  StateValueAtInitialization/2 -> Integration Logic/3
  dxdt/State -> StateValueAtInitialization/3
  InternalICDXDT/1(dx0Internal) -> dxdt/3

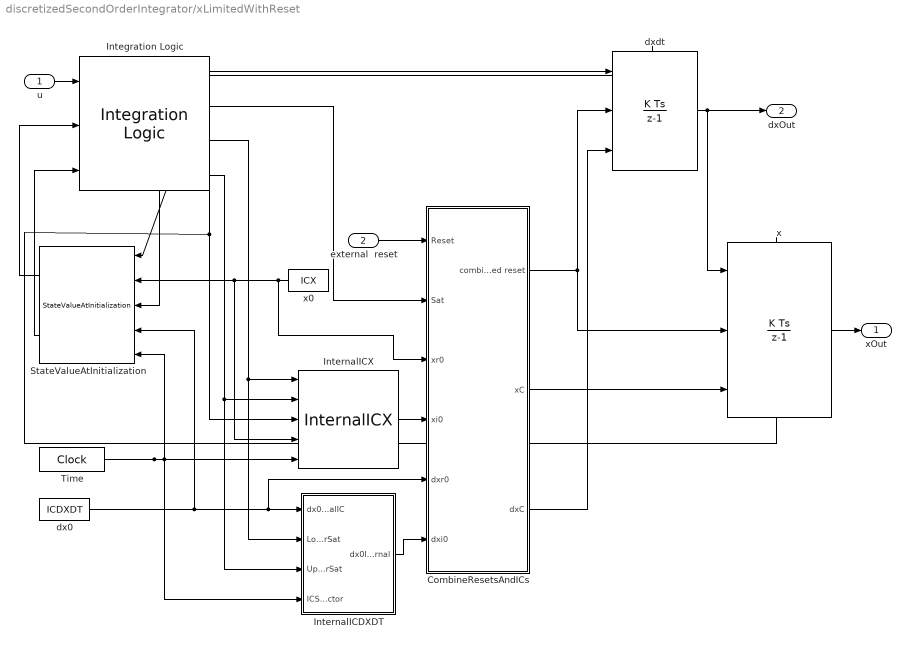
== system discretizedSecondOrderIntegrator/xLimitedWithReset ==
  u : Inport
  external  reset : Inport  Port=2
  CombineResetsAndICs : Subsystem
  Integration Logic : discretizedSecondOrderIntegrator/Integration Logic  SystemSampleTime=-1
  InternalICDXDT : Subsystem  mask{ReinitDXDTwhenXreachesSaturation=off}
      mask prompts: ReinitDXDTwhenXreachesSaturation "Reinitialize dx/dt when x reaches saturation"
      mask init:
      | if strcmp(get_param(gcb, 'ReinitDXDTwhenXreachesSaturation'), 'on')
      |      set_param([gcb '/ReinitializationFlag'], 'Value','1');
      | else
      |     set_param([gcb '/ReinitializationFlag'], 'Value','0');
      | end
  InternalICX : discretizedSecondOrderIntegrator/InternalICX  SystemSampleTime=-1
  StateValueAtInitialization : discretizedSecondOrderIntegrator/StateValueAtInitialization  SystemSampleTime=-1
  Time : DigitalClock  SampleTime=SampleTime
  dx0 : Constant  Value=ICDXDT
  dxdt : DiscreteIntegrator  gainval=GainValue  ExternalReset=rising  InitialConditionSource=external  InitialCondition=ICDXDT  SampleTime=SampleTime  OutDataType=fixdt(1, 16)  OutScaling=2^0  UpperSaturationLimit=UpperLimitDXDT  LowerSaturationLimit=LowerLimitDXDT  ShowStatePort=on  ICPrevOutput=DiscIntNeverNeededParam  ICPrevScaledInput=DiscIntNeverNeededParam
  x : DiscreteIntegrator  gainval=GainValue  ExternalReset=rising  InitialConditionSource=external  InitialCondition=ICX  SampleTime=SampleTime  OutDataType=fixdt(1, 16)  OutScaling=2^0  LimitOutput=on  UpperSaturationLimit=UpperLimitX  LowerSaturationLimit=LowerLimitX  ShowStatePort=on  ICPrevOutput=DiscIntNeverNeededParam  ICPrevScaledInput=DiscIntNeverNeededParam
  x0 : Constant  Value=ICX
  xOut : Outport
  dxOut : Outport  Port=2
  wires:
  Integration Logic/1 -> dxdt/1
  u/1 -> Integration Logic/1
  x/1 -> xOut/1
  dxdt/1 -> dxOut/1, x/1
  x/State -> InternalICX/3, StateValueAtInitialization/1
  Integration Logic/3 -> InternalICX/1, InternalICDXDT/2(LowerSat)
  Integration Logic/4 -> InternalICX/2, InternalICDXDT/3(UpperSat)
  external  reset/1 -> CombineResetsAndICs/1("Reset ")
  Integration Logic/2 -> CombineResetsAndICs/2(Sat)
  dx0/1 -> CombineResetsAndICs/5(dxr0), InternalICDXDT/1(dx0ExternalIC), StateValueAtInitialization/4
  InternalICX/1 -> CombineResetsAndICs/4(xi0)
  CombineResetsAndICs/2(xC) -> x/3
  CombineResetsAndICs/1(combined reset) -> dxdt/2, x/2
  Time/1 -> InternalICX/5, StateValueAtInitialization/5, InternalICDXDT/4(ICSelector)
  StateValueAtInitialization/1 -> Integration Logic/2
  StateValueAtInitialization/2 -> Integration Logic/3
  dxdt/State -> StateValueAtInitialization/3
  x0/1 -> StateValueAtInitialization/2, InternalICX/4, CombineResetsAndICs/3(xr0)
  CombineResetsAndICs/3(dxC) -> dxdt/3
  InternalICDXDT/1(dx0Internal) -> CombineResetsAndICs/6(dxi0)

== system discretizedSecondOrderIntegrator/CombineResetsAndICs/ExternalResetModifier ==
  In1 : Inport
  risingE : discretizedSecondOrderIntegrator/risingE  SystemSampleTime=-1
  Out1 : Outport
  wires:
  In1/1 -> risingE/1
  risingE/1 -> Out1/1

== system discretizedSecondOrderIntegrator/CombineResetsAndICs/InternalResetModifier ==
  In1 : Inport
  risingI : discretizedSecondOrderIntegrator/risingI  SystemSampleTime=-1
  Out1 : Outport
  wires:
  In1/1 -> risingI/1
  risingI/1 -> Out1/1

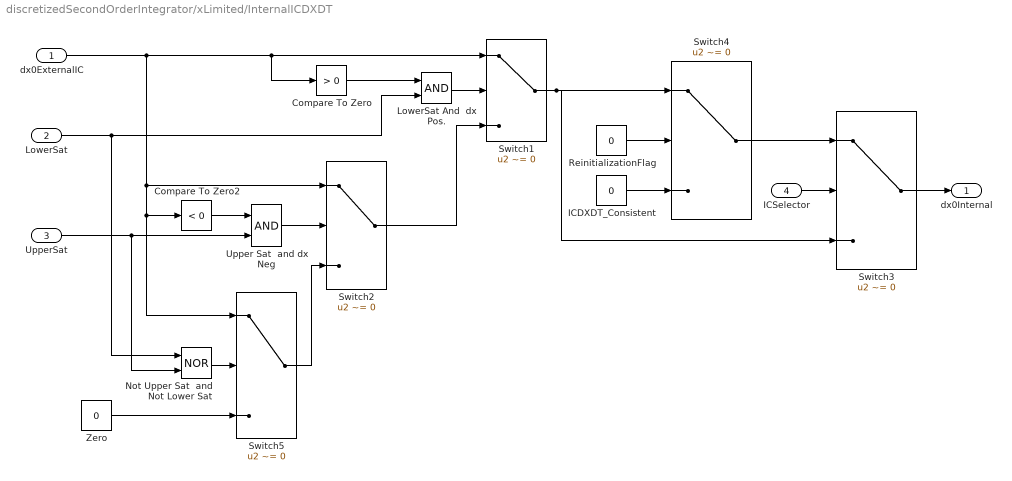
== system discretizedSecondOrderIntegrator/xLimited/InternalICDXDT ==
  dx0ExternalIC : Inport
  LowerSat : Inport  Port=2
  UpperSat : Inport  Port=3
  ICSelector : Inport  Port=4
  Compare To Zero : simulink/Logic and Bit Operations/Compare To Zero  SystemSampleTime=-1  relop=>  LogicOutDataTypeMode=boolean
  Compare To Zero2 : simulink/Logic and Bit Operations/Compare To Zero  SystemSampleTime=-1  relop=<  LogicOutDataTypeMode=boolean
  ICDXDT_Consistent : Constant  Value=0  OutDataType=fixdt(1, 16)  OutScaling=2^0
  LowerSat And  dx Pos. : Logic  AllPortsSameDT=off  OutDataTypeMode=boolean  LogicDataType=fixdt(0, 8)  OutDataTypeStr=boolean
  Not Upper Sat  and Not Lower Sat : Logic  Operator=NOR  AllPortsSameDT=off  OutDataTypeMode=boolean  LogicDataType=fixdt(0, 8)  OutDataTypeStr=boolean
  ReinitializationFlag : Constant  Value=0  OutDataType=fixdt(1, 16)  OutScaling=2^0
  Switch{1..5} (5 alike) : Switch  Criteria=u2 ~= 0  OutDataType=fixdt(1, 16)  OutScaling=2^0
  Upper Sat  and dx Neg : Logic  AllPortsSameDT=off  OutDataTypeMode=boolean  LogicDataType=fixdt(0, 8)  OutDataTypeStr=boolean
  Zero : Constant  Value=0  OutDataType=fixdt(1, 16)  OutScaling=2^0
  dx0Internal : Outport
  wires:
  Not Upper Sat  and Not Lower Sat/1 -> Switch5/2
  Switch5/1 -> Switch2/3
  Zero/1 -> Switch5/3
  Switch4/1 -> Switch3/1
  dx0ExternalIC/1 -> Switch1/1, Compare To Zero/1, Compare To Zero2/1, Switch5/1, Switch2/1
  ICDXDT_Consistent/1 -> Switch4/3
  ReinitializationFlag/1 -> Switch4/2
  Switch3/1 -> dx0Internal/1
  Switch1/1 -> Switch3/3, Switch4/1
  Compare To Zero2/1 -> Upper Sat  and dx Neg/1
  UpperSat/1 -> Not Upper Sat  and Not Lower Sat/2, Upper Sat  and dx Neg/2
  Switch2/1 -> Switch1/3
  LowerSat/1 -> Not Upper Sat  and Not Lower Sat/1, LowerSat And  dx Pos./2
  Compare To Zero/1 -> LowerSat And  dx Pos./1
  LowerSat And  dx Pos./1 -> Switch1/2
  Upper Sat  and dx Neg/1 -> Switch2/2
  ICSelector/1 -> Switch3/2

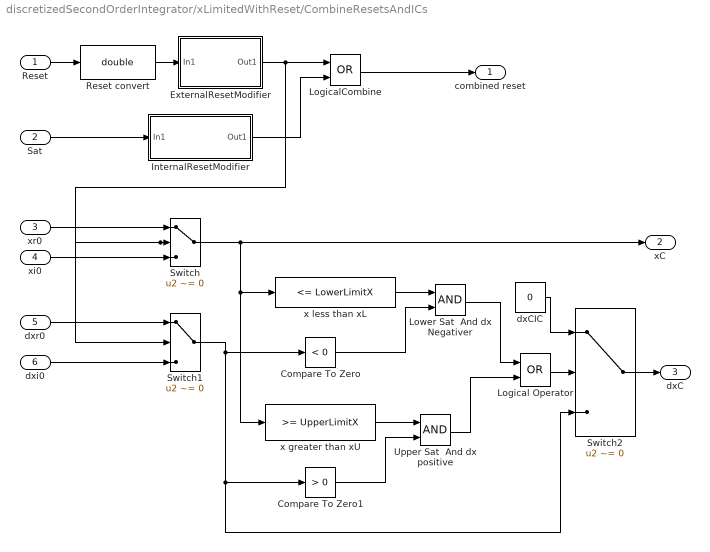
== system discretizedSecondOrderIntegrator/xLimitedWithReset/CombineResetsAndICs ==
  "Reset " : Inport  OutDataType=fixdt(1, 16)  OutScaling=2^0
  Sat : Inport  Port=2  OutDataType=fixdt(1, 16)  OutScaling=2^0
  xr0 : Inport  Port=3  OutDataType=fixdt(1, 16)  OutScaling=2^0
  xi0 : Inport  Port=4  OutDataType=fixdt(1, 16)  OutScaling=2^0
  dxr0 : Inport  Port=5  OutDataType=fixdt(1, 16)  OutScaling=2^0
  dxi0 : Inport  Port=6  OutDataType=fixdt(1, 16)  OutScaling=2^0
  Compare To Zero : simulink/Logic and Bit Operations/Compare To Zero  SystemSampleTime=-1  relop=<  LogicOutDataTypeMode=boolean
  Compare To Zero1 : simulink/Logic and Bit Operations/Compare To Zero  SystemSampleTime=-1  relop=>  LogicOutDataTypeMode=boolean
  ExternalResetModifier : Subsystem  BlockChoice=risingE
      settings: AttributesFormatString=%<BlockChoice>  TemplateBlock=discretizedSecondOrderIntegrator/External Reset Modifier  MemberBlocks=eitherE,fallingE,risingE
  InternalResetModifier : Subsystem  BlockChoice=risingI
      settings: AttributesFormatString=%<BlockChoice>  TemplateBlock=discretizedSecondOrderIntegrator/Internal Reset Modifer  MemberBlocks=eitherI,fallingI,risingI
  Logical Operator : Logic  Operator=OR  AllPortsSameDT=off  OutDataTypeMode=boolean  LogicDataType=fixdt(0, 8)  OutDataTypeStr=boolean
  LogicalCombine : Logic  Operator=OR  AllPortsSameDT=off  OutDataTypeMode=boolean  LogicDataType=fixdt(0, 8)  OutDataTypeStr=boolean
  Lower Sat  And dx Negativer : Logic  AllPortsSameDT=off  OutDataTypeMode=boolean  LogicDataType=fixdt(0, 8)  OutDataTypeStr=boolean
  Reset convert : DataTypeConversion  OutDataTypeMode=double  OutDataType=fixdt(1, 16)  OutScaling=2^0  OutDataTypeStr=double
  Switch : Switch  Criteria=u2 ~= 0  OutDataType=fixdt(1, 16)  OutScaling=2^0
  Switch1 : Switch  Criteria=u2 ~= 0  OutDataType=fixdt(1, 16)  OutScaling=2^0
  Switch2 : Switch  Criteria=u2 ~= 0  OutDataType=fixdt(1, 16)  OutScaling=2^0
  Upper Sat  And dx positive : Logic  AllPortsSameDT=off  OutDataTypeMode=boolean  LogicDataType=fixdt(0, 8)  OutDataTypeStr=boolean
  dxCIC : Constant  Value=0  OutDataType=fixdt(1, 16)  OutScaling=2^0
  x greater than xU : simulink/Logic and Bit Operations/Compare To Constant  SystemSampleTime=-1  relop=>=  const=UpperLimitX  LogicOutDataTypeMode=boolean
  x less than xL : simulink/Logic and Bit Operations/Compare To Constant  SystemSampleTime=-1  relop=<=  const=LowerLimitX  LogicOutDataTypeMode=boolean
  combined reset : Outport  OutDataType=fixdt(1, 16)  OutScaling=2^0
  xC : Outport  Port=2  OutDataType=fixdt(1, 16)  OutScaling=2^0
  dxC : Outport  Port=3  OutDataType=fixdt(1, 16)  OutScaling=2^0
  wires:
  InternalResetModifier/1(Out1) -> LogicalCombine/2
  Compare To Zero/1 -> Lower Sat  And dx Negativer/2
  Compare To Zero1/1 -> Upper Sat  And dx positive/2
  x greater than xU/1 -> Upper Sat  And dx positive/1
  x less than xL/1 -> Lower Sat  And dx Negativer/1
  Upper Sat  And dx positive/1 -> Logical Operator/2
  Lower Sat  And dx Negativer/1 -> Logical Operator/1
  dxCIC/1 -> Switch2/1
  Switch/1 -> x greater than xU/1, x less than xL/1, xC/1
  Switch1/1 -> Compare To Zero/1, Compare To Zero1/1, Switch2/3
  Switch2/1 -> dxC/1
  Logical Operator/1 -> Switch2/2
  xi0/1 -> Switch/3
  xr0/1 -> Switch/1
  Reset convert/1 -> ExternalResetModifier/1(In1)
  ExternalResetModifier/1(Out1) -> LogicalCombine/1, Switch/2, Switch1/2
  "Reset "/1 -> Reset convert/1
  LogicalCombine/1 -> combined reset/1
  dxr0/1 -> Switch1/1
  dxi0/1 -> Switch1/3
  Sat/1 -> InternalResetModifier/1(In1)

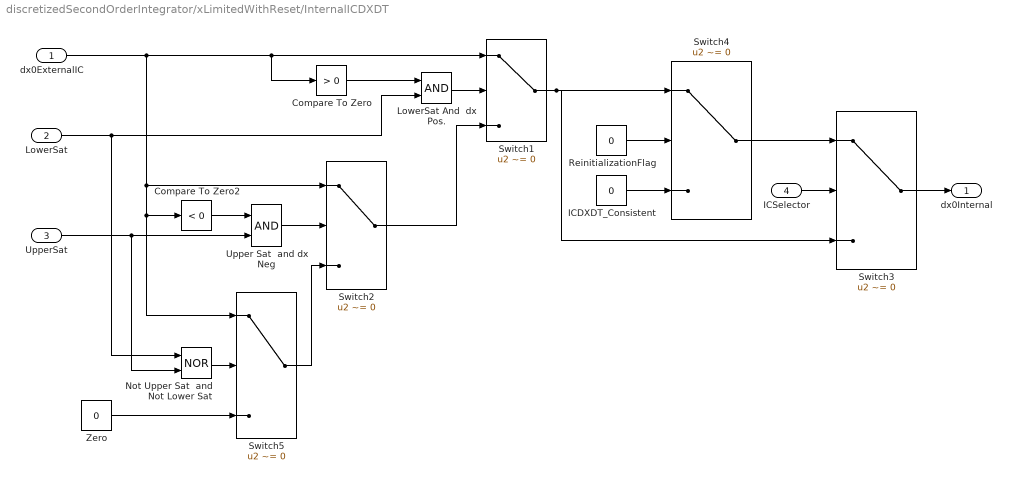
== system discretizedSecondOrderIntegrator/xLimitedWithReset/InternalICDXDT ==
  dx0ExternalIC : Inport
  LowerSat : Inport  Port=2
  UpperSat : Inport  Port=3
  ICSelector : Inport  Port=4
  Compare To Zero : simulink/Logic and Bit Operations/Compare To Zero  SystemSampleTime=-1  relop=>  LogicOutDataTypeMode=boolean
  Compare To Zero2 : simulink/Logic and Bit Operations/Compare To Zero  SystemSampleTime=-1  relop=<  LogicOutDataTypeMode=boolean
  ICDXDT_Consistent : Constant  Value=0  OutDataType=fixdt(1, 16)  OutScaling=2^0
  LowerSat And  dx Pos. : Logic  AllPortsSameDT=off  OutDataTypeMode=boolean  LogicDataType=fixdt(0, 8)  OutDataTypeStr=boolean
  Not Upper Sat  and Not Lower Sat : Logic  Operator=NOR  AllPortsSameDT=off  OutDataTypeMode=boolean  LogicDataType=fixdt(0, 8)  OutDataTypeStr=boolean
  ReinitializationFlag : Constant  Value=0  OutDataType=fixdt(1, 16)  OutScaling=2^0
  Switch{1..5} (5 alike) : Switch  Criteria=u2 ~= 0  OutDataType=fixdt(1, 16)  OutScaling=2^0
  Upper Sat  and dx Neg : Logic  AllPortsSameDT=off  OutDataTypeMode=boolean  LogicDataType=fixdt(0, 8)  OutDataTypeStr=boolean
  Zero : Constant  Value=0  OutDataType=fixdt(1, 16)  OutScaling=2^0
  dx0Internal : Outport
  wires:
  Not Upper Sat  and Not Lower Sat/1 -> Switch5/2
  Switch5/1 -> Switch2/3
  Zero/1 -> Switch5/3
  Switch4/1 -> Switch3/1
  dx0ExternalIC/1 -> Switch1/1, Compare To Zero/1, Compare To Zero2/1, Switch5/1, Switch2/1
  ICDXDT_Consistent/1 -> Switch4/3
  ReinitializationFlag/1 -> Switch4/2
  Switch3/1 -> dx0Internal/1
  Switch1/1 -> Switch3/3, Switch4/1
  Compare To Zero2/1 -> Upper Sat  and dx Neg/1
  UpperSat/1 -> Not Upper Sat  and Not Lower Sat/2, Upper Sat  and dx Neg/2
  Switch2/1 -> Switch1/3
  LowerSat/1 -> Not Upper Sat  and Not Lower Sat/1, LowerSat And  dx Pos./2
  Compare To Zero/1 -> LowerSat And  dx Pos./1
  LowerSat And  dx Pos./1 -> Switch1/2
  Upper Sat  and dx Neg/1 -> Switch2/2
  ICSelector/1 -> Switch3/2

== system discretizedSecondOrderIntegrator/xLimitedWithReset/CombineResetsAndICs/ExternalResetModifier ==
  In1 : Inport
  risingE : discretizedSecondOrderIntegrator/risingE  SystemSampleTime=-1
  Out1 : Outport
  wires:
  In1/1 -> risingE/1
  risingE/1 -> Out1/1

== system discretizedSecondOrderIntegrator/xLimitedWithReset/CombineResetsAndICs/InternalResetModifier ==
  In1 : Inport
  risingI : discretizedSecondOrderIntegrator/risingI  SystemSampleTime=-1
  Out1 : Outport
  wires:
  In1/1 -> risingI/1
  risingI/1 -> Out1/1
